simulink model "PILnewH"  (R2021a)
settings: Solver=FixedStepAuto  StartTime=0.0  StopTime=41.24  FixedStep=0.001  RelTol=1e-3  EnableMultiTasking=on
values from neighbouring files (symbols this model uses):
  den_lpf_d = den_lpf20    [Mainframe_init.m]    (also in load_autopilot.m)
  Emulated_FCC_IO_Delay = 7    [Mainframe_init.m]
  Enable_Gyros = 0    [Mainframe_init.m]
  Enable_INS = 0    [Mainframe_init.m]
  num_lpf_d = num_lpf20    [Mainframe_init.m]    (also in load_autopilot.m)
undefined symbols (not defined in the file or in its folder): act_dmp, act_omega, Actuator, Aerodynamics, aMode, Autopilot, AUX, c_b_WGS, c_be, c_flat, c_grav, c_h_geop0, c_h_geope, c_pa0, c_pe, c_r0, c_rot, c_rsma, c_Tmp0, d_siB_0, d_siB_max, d_siB_min, dd_siB_max, dd_siB_min, dev, DiscIntNeverNeededParam, e_pa, e_Tmp, Earth, fin_maxrate, flag_I_act_switch, flag_I_aero_switch, flag_I_flat, flag_I_gravity_switch, flag_I_rot, hcr, HIL_Data, JMMM_0, JMMM_e, JSPB_e, lat_0, lon_0, Mass_Props, mB_0, mM_0, mM_e, National_Instruments, pBII_0, PCIe, pMPB, pNPB, propellant_kg, prp_FBPB, prp_mdot, prp_T, pSPB, pwm_output1, qEG_0, qIB_0, qIE_0 ... (+29)
libraries: simulink x31, simulink_extras x24, aerolibcommonsys x4, px4lib x2, custom_blocks x1, pil_lib x1, aerolibtransform2 x1, sldrtlib x1, aerolibnav x1
(part 8 of 15)

== system PILnewH/Non-linear Flight Dynamic Model/GRM_Airframe/motion_kinematics/calc_motion_kinematics/earth_rotation/quaternion_integration ==
  wEIE : Inport
  Constant8 : Constant  Value=qIE_0
  Subsystem1 : Subsystem
  T12_from_q12 : Subsystem
      mask help: Transforms a quaternion into a Direction Cosine Matrix
      mask Help:
      | Name:
      | 
      |     T12_from_q12
      | 
      | Description:
      | 
      |     This block implements the transformation of a quaternion into the
      |     corresponding direction cosine matrix DCM.
      | 
      | Inputs  [size] [data type] [unit]:
      | 
      |     quaternion q12 [4] [double] [-]
      | 
      | Outputs  [size] [data type] [unit]:
      | 
      |     direction cosine matrix T12  [3x3] [double] [-]
      mask Display:
      | %port_label('input', 1, 'q12')
      | %port_label('output', 1, 'T12')
      | disp('q \rightarrow DCM','texmode','on')
  integration_eom : Integrator  InitialConditionSource=external
  qIE : Outport  VectorParamsAs1DForOutWhenUnconnected=off
  TIE : Outport  Port=2  VectorParamsAs1DForOutWhenUnconnected=off
  wires:
  Subsystem1/1(d_qIE) -> integration_eom/1
  integration_eom/1 -> qIE/1, Subsystem1/2(qIE), T12_from_q12/1(q12)  "qIE"
  wEIE/1 -> Subsystem1/1(wEIE)
  T12_from_q12/1(T12) -> TIE/1  "TIE"
  Constant8/1 -> integration_eom/2

== system PILnewH/Non-linear Flight Dynamic Model/GRM_Airframe/motion_kinematics/calc_motion_kinematics/earth_rotation/quaternion_integration1 ==
  wGEG : Inport
  Constant8 : Constant  Value=qEG_0
  Subsystem1 : Subsystem
  T12_from_q12 : Subsystem
      mask help: Transforms a quaternion into a Direction Cosine Matrix
      mask Help:
      | Name:
      | 
      |     T12_from_q12
      | 
      | Description:
      | 
      |     This block implements the transformation of a quaternion into the
      |     corresponding direction cosine matrix DCM.
      | 
      | Inputs  [size] [data type] [unit]:
      | 
      |     quaternion q12 [4] [double] [-]
      | 
      | Outputs  [size] [data type] [unit]:
      | 
      |     direction cosine matrix T12  [3x3] [double] [-]
      mask Display:
      | %port_label('input', 1, 'q12')
      | %port_label('output', 1, 'T12')
      | disp('q \rightarrow DCM','texmode','on')
  integration_eom : Integrator  InitialConditionSource=external
  qEG : Outport  VectorParamsAs1DForOutWhenUnconnected=off
  TEG : Outport  Port=2  VectorParamsAs1DForOutWhenUnconnected=off
  wires:
  Constant8/1 -> integration_eom/2
  T12_from_q12/1(T12) -> TEG/1  "TEG"
  wGEG/1 -> Subsystem1/1(wGEG)
  integration_eom/1 -> T12_from_q12/1(q12), Subsystem1/2(qEG), qEG/1  "qEG"
  Subsystem1/1(d_qEG) -> integration_eom/1

== system PILnewH/Non-linear Flight Dynamic Model/GRM_Airframe/motion_kinematics/calc_motion_kinematics/earth_rotation/transport_rate ==
  lat : Inport
  lon : Inport  Port=2
  Constant8 : Constant  Value=0
  Constant9 : Constant  Value=flag_I_flat
  Derivative : Derivative  CoefficientInTFapproximation=1
  Derivative1 : Derivative  CoefficientInTFapproximation=1
  Gain1 : Gain  Gain=-1
  Gain2 : Gain  Gain=-1
  Product : Product
  Product1 : Product
  Switch : Switch  Criteria=u2 > Threshold
  Trigonometric Function : Trigonometry
  Trigonometric Function1 : Trigonometry  Operator=cos
  Vector Concatenate : Concatenate  NumInputs=3
  Vector Concatenate1 : Concatenate  NumInputs=3
  wEGG : Outport  VectorParamsAs1DForOutWhenUnconnected=off
  wires:
  Derivative/1 -> Gain1/1
  Trigonometric Function/1 -> Product/1
  lat/1 -> Trigonometric Function1/1, Derivative/1, Trigonometric Function/1
  Derivative1/1 -> Product1/1, Product/2
  Product/1 -> Gain2/1
  Gain2/1 -> Vector Concatenate/3
  Gain1/1 -> Vector Concatenate/2
  Product1/1 -> Vector Concatenate/1
  Trigonometric Function1/1 -> Product1/2
  lon/1 -> Derivative1/1
  Vector Concatenate/1 -> Switch/3  "wEGG"
  Constant9/1 -> Switch/2
  Vector Concatenate1/1 -> Switch/1  "wEGG"
  Constant8/1 -> Vector Concatenate1/1, Vector Concatenate1/3, Vector Concatenate1/2
  Switch/1 -> wEGG/1  "wEGG"

== system PILnewH/Non-linear Flight Dynamic Model/GRM_Airframe/propulsion/prp_uncertainty/3_rot_mat/1. Rotation x-Achse ==
  alpha1 : Inport
  Constant : Constant
  Constant{1..2,7..8} (4 alike) : Constant  Value=0
  Gain : Gain  Gain=-1
  Matrix Concatenate : Concatenate  NumInputs=3  Mode=Multidimensional array  ConcatenateDimension=2
  Mux : Mux  Inputs=3
  Mux1 : Mux  Inputs=3
  Mux2 : Mux  Inputs=3
  Trigonometric Function : Trigonometry  Operator=cos
  Trigonometric Function1 : Trigonometry
  Trigonometric Function2 : Trigonometry
  Trigonometric Function3 : Trigonometry  Operator=cos
  1Rot_Matrix_x : Outport  VectorParamsAs1DForOutWhenUnconnected=off
  wires:
  Gain/1 -> Mux1/3
  alpha1/1 -> Trigonometric Function2/1, Trigonometric Function/1, Trigonometric Function1/1, Trigonometric Function3/1
  Constant/1 -> Mux/1
  Constant1/1 -> Mux/2
  Constant2/1 -> Mux/3
  Constant8/1 -> Mux1/1
  Trigonometric Function/1 -> Mux1/2
  Trigonometric Function2/1 -> Gain/1
  Constant7/1 -> Mux2/1
  Trigonometric Function1/1 -> Mux2/2
  Trigonometric Function3/1 -> Mux2/3
  Mux/1 -> Matrix Concatenate/1
  Mux1/1 -> Matrix Concatenate/2
  Mux2/1 -> Matrix Concatenate/3
  Matrix Concatenate/1 -> 1Rot_Matrix_x/1

== system PILnewH/Non-linear Flight Dynamic Model/GRM_Airframe/propulsion/prp_uncertainty/3_rot_mat/1. Rotation y-Achse ==
  alpha1 : Inport
  Constant{,2,7..8} (4 alike) : Constant  Value=0
  Constant1 : Constant
  Gain1 : Gain  Gain=-1
  Matrix Concatenate : Concatenate  NumInputs=3  Mode=Multidimensional array  ConcatenateDimension=2
  Mux : Mux  Inputs=3
  Mux1 : Mux  Inputs=3
  Mux2 : Mux  Inputs=3
  Trigonometric Function : Trigonometry  Operator=cos
  Trigonometric Function1 : Trigonometry
  Trigonometric Function2 : Trigonometry
  Trigonometric Function3 : Trigonometry  Operator=cos
  1Rot_Matrix_y : Outport  VectorParamsAs1DForOutWhenUnconnected=off
  wires:
  Gain1/1 -> Mux2/1
  Mux2/1 -> Matrix Concatenate/3
  Mux1/1 -> Matrix Concatenate/2
  Mux/1 -> Matrix Concatenate/1
  Trigonometric Function3/1 -> Mux2/3
  Trigonometric Function1/1 -> Gain1/1
  Constant2/1 -> Mux1/3
  Constant1/1 -> Mux1/2
  Constant/1 -> Mux1/1
  alpha1/1 -> Trigonometric Function1/1, Trigonometric Function3/1, Trigonometric Function2/1, Trigonometric Function/1
  Constant8/1 -> Mux/2
  Trigonometric Function/1 -> Mux/1
  Trigonometric Function2/1 -> Mux/3
  Constant7/1 -> Mux2/2
  Matrix Concatenate/1 -> 1Rot_Matrix_y/1

== system PILnewH/Non-linear Flight Dynamic Model/GRM_Airframe/propulsion/prp_uncertainty/3_rot_mat/1. Rotation z-Achse ==
  alpha1 : Inport
  Constant{4,7..8,10} (4 alike) : Constant  Value=0
  Constant11 : Constant
  Gain : Gain  Gain=-1
  Matrix Concatenate : Concatenate  NumInputs=3  Mode=Multidimensional array  ConcatenateDimension=2
  Mux : Mux  Inputs=3
  Mux1 : Mux  Inputs=3
  Mux2 : Mux  Inputs=3
  Trigonometric Function : Trigonometry  Operator=cos
  Trigonometric Function1 : Trigonometry
  Trigonometric Function3 : Trigonometry  Operator=cos
  Trigonometric Function4 : Trigonometry
  1Rot_Matrix_z : Outport  VectorParamsAs1DForOutWhenUnconnected=off
  wires:
  Gain/1 -> Mux/2
  Trigonometric Function/1 -> Mux1/2
  Mux/1 -> Matrix Concatenate/1
  Mux1/1 -> Matrix Concatenate/2
  Mux2/1 -> Matrix Concatenate/3
  Trigonometric Function1/1 -> Mux1/1
  Constant7/1 -> Mux1/3
  Constant4/1 -> Mux2/1
  Constant10/1 -> Mux2/2
  Constant11/1 -> Mux2/3
  Trigonometric Function3/1 -> Mux/1
  Trigonometric Function4/1 -> Gain/1
  Constant8/1 -> Mux/3
  Matrix Concatenate/1 -> 1Rot_Matrix_z/1
  alpha1/1 -> Trigonometric Function3/1, Trigonometric Function4/1, Trigonometric Function/1, Trigonometric Function1/1

== system PILnewH/Non-linear Flight Dynamic Model/GRM_Airframe/propulsion/prp_uncertainty/3_rot_mat/2. Rotation x-Achse ==
  alpha2 : Inport
  Constant : Constant
  Constant{1..2,7..8} (4 alike) : Constant  Value=0
  Gain : Gain  Gain=-1
  Matrix Concatenate : Concatenate  NumInputs=3  Mode=Multidimensional array  ConcatenateDimension=2
  Mux : Mux  Inputs=3
  Mux1 : Mux  Inputs=3
  Mux2 : Mux  Inputs=3
  Trigonometric Function : Trigonometry  Operator=cos
  Trigonometric Function1 : Trigonometry
  Trigonometric Function2 : Trigonometry
  Trigonometric Function3 : Trigonometry  Operator=cos
  2Rot_Matrix_x : Outport  VectorParamsAs1DForOutWhenUnconnected=off
  wires:
  Gain/1 -> Mux1/3
  alpha2/1 -> Trigonometric Function2/1, Trigonometric Function/1, Trigonometric Function1/1, Trigonometric Function3/1
  Constant/1 -> Mux/1
  Constant1/1 -> Mux/2
  Constant2/1 -> Mux/3
  Constant8/1 -> Mux1/1
  Trigonometric Function/1 -> Mux1/2
  Trigonometric Function2/1 -> Gain/1
  Constant7/1 -> Mux2/1
  Trigonometric Function1/1 -> Mux2/2
  Trigonometric Function3/1 -> Mux2/3
  Mux/1 -> Matrix Concatenate/1
  Mux1/1 -> Matrix Concatenate/2
  Mux2/1 -> Matrix Concatenate/3
  Matrix Concatenate/1 -> 2Rot_Matrix_x/1

== system PILnewH/Non-linear Flight Dynamic Model/GRM_Airframe/propulsion/prp_uncertainty/3_rot_mat/2. Rotation y-Achse ==
  alpha2 : Inport
  Constant{,2,7..8} (4 alike) : Constant  Value=0
  Constant1 : Constant
  Gain1 : Gain  Gain=-1
  Matrix Concatenate : Concatenate  NumInputs=3  Mode=Multidimensional array  ConcatenateDimension=2
  Mux : Mux  Inputs=3
  Mux1 : Mux  Inputs=3
  Mux2 : Mux  Inputs=3
  Trigonometric Function : Trigonometry  Operator=cos
  Trigonometric Function1 : Trigonometry
  Trigonometric Function2 : Trigonometry
  Trigonometric Function3 : Trigonometry  Operator=cos
  2Rot_Matrix_y : Outport  VectorParamsAs1DForOutWhenUnconnected=off
  wires:
  Gain1/1 -> Mux2/1
  Mux2/1 -> Matrix Concatenate/3
  Mux1/1 -> Matrix Concatenate/2
  Mux/1 -> Matrix Concatenate/1
  Trigonometric Function3/1 -> Mux2/3
  Trigonometric Function1/1 -> Gain1/1
  Constant2/1 -> Mux1/3
  Constant1/1 -> Mux1/2
  Constant/1 -> Mux1/1
  alpha2/1 -> Trigonometric Function1/1, Trigonometric Function3/1, Trigonometric Function2/1, Trigonometric Function/1
  Constant8/1 -> Mux/2
  Trigonometric Function/1 -> Mux/1
  Trigonometric Function2/1 -> Mux/3
  Constant7/1 -> Mux2/2
  Matrix Concatenate/1 -> 2Rot_Matrix_y/1

== system PILnewH/Non-linear Flight Dynamic Model/GRM_Airframe/propulsion/prp_uncertainty/3_rot_mat/2. Rotation z-Achse ==
  alpha2 : Inport
  Constant{4,7..8,10} (4 alike) : Constant  Value=0
  Constant11 : Constant
  Gain : Gain  Gain=-1
  Matrix Concatenate : Concatenate  NumInputs=3  Mode=Multidimensional array  ConcatenateDimension=2
  Mux : Mux  Inputs=3
  Mux1 : Mux  Inputs=3
  Mux2 : Mux  Inputs=3
  Trigonometric Function : Trigonometry  Operator=cos
  Trigonometric Function1 : Trigonometry
  Trigonometric Function3 : Trigonometry  Operator=cos
  Trigonometric Function4 : Trigonometry
  2Rot_Matrix_z : Outport  VectorParamsAs1DForOutWhenUnconnected=off
  wires:
  Gain/1 -> Mux/2
  Trigonometric Function/1 -> Mux1/2
  Mux/1 -> Matrix Concatenate/1
  Mux1/1 -> Matrix Concatenate/2
  Mux2/1 -> Matrix Concatenate/3
  Trigonometric Function1/1 -> Mux1/1
  Constant7/1 -> Mux1/3
  Constant4/1 -> Mux2/1
  Constant10/1 -> Mux2/2
  Constant11/1 -> Mux2/3
  Trigonometric Function3/1 -> Mux/1
  Trigonometric Function4/1 -> Gain/1
  Constant8/1 -> Mux/3
  Matrix Concatenate/1 -> 2Rot_Matrix_z/1
  alpha2/1 -> Trigonometric Function3/1, Trigonometric Function4/1, Trigonometric Function/1, Trigonometric Function1/1

== system PILnewH/Non-linear Flight Dynamic Model/GRM_Airframe/propulsion/prp_uncertainty/3_rot_mat/3. Rotation x-Achse ==
  alpha3 : Inport
  Constant : Constant
  Constant{1..2,7..8} (4 alike) : Constant  Value=0
  Gain : Gain  Gain=-1
  Matrix Concatenate : Concatenate  NumInputs=3  Mode=Multidimensional array  ConcatenateDimension=2
  Mux : Mux  Inputs=3
  Mux1 : Mux  Inputs=3
  Mux2 : Mux  Inputs=3
  Trigonometric Function : Trigonometry  Operator=cos
  Trigonometric Function1 : Trigonometry
  Trigonometric Function2 : Trigonometry
  Trigonometric Function3 : Trigonometry  Operator=cos
  3Rot_Matrix_x : Outport  VectorParamsAs1DForOutWhenUnconnected=off
  wires:
  Gain/1 -> Mux1/3
  alpha3/1 -> Trigonometric Function2/1, Trigonometric Function/1, Trigonometric Function1/1, Trigonometric Function3/1
  Constant/1 -> Mux/1
  Constant1/1 -> Mux/2
  Constant2/1 -> Mux/3
  Constant8/1 -> Mux1/1
  Trigonometric Function/1 -> Mux1/2
  Trigonometric Function2/1 -> Gain/1
  Constant7/1 -> Mux2/1
  Trigonometric Function1/1 -> Mux2/2
  Trigonometric Function3/1 -> Mux2/3
  Mux/1 -> Matrix Concatenate/1
  Mux1/1 -> Matrix Concatenate/2
  Mux2/1 -> Matrix Concatenate/3
  Matrix Concatenate/1 -> 3Rot_Matrix_x/1

== system PILnewH/Non-linear Flight Dynamic Model/GRM_Airframe/propulsion/prp_uncertainty/3_rot_mat/3. Rotation y-Achse ==
  alpha3 : Inport
  Constant{,2,7..8} (4 alike) : Constant  Value=0
  Constant1 : Constant
  Gain1 : Gain  Gain=-1
  Matrix Concatenate : Concatenate  NumInputs=3  Mode=Multidimensional array  ConcatenateDimension=2
  Mux : Mux  Inputs=3
  Mux1 : Mux  Inputs=3
  Mux2 : Mux  Inputs=3
  Trigonometric Function : Trigonometry  Operator=cos
  Trigonometric Function1 : Trigonometry
  Trigonometric Function2 : Trigonometry
  Trigonometric Function3 : Trigonometry  Operator=cos
  3Rot_Matrix_y : Outport  VectorParamsAs1DForOutWhenUnconnected=off
  wires:
  Gain1/1 -> Mux2/1
  Mux2/1 -> Matrix Concatenate/3
  Mux1/1 -> Matrix Concatenate/2
  Mux/1 -> Matrix Concatenate/1
  Trigonometric Function3/1 -> Mux2/3
  Trigonometric Function1/1 -> Gain1/1
  Constant2/1 -> Mux1/3
  Constant1/1 -> Mux1/2
  Constant/1 -> Mux1/1
  alpha3/1 -> Trigonometric Function1/1, Trigonometric Function3/1, Trigonometric Function2/1, Trigonometric Function/1
  Constant8/1 -> Mux/2
  Trigonometric Function/1 -> Mux/1
  Trigonometric Function2/1 -> Mux/3
  Constant7/1 -> Mux2/2
  Matrix Concatenate/1 -> 3Rot_Matrix_y/1

== system PILnewH/Non-linear Flight Dynamic Model/GRM_Airframe/propulsion/prp_uncertainty/3_rot_mat/3. Rotation z-Achse ==
  alpha3 : Inport
  Constant{4,7..8,10} (4 alike) : Constant  Value=0
  Constant11 : Constant
  Gain : Gain  Gain=-1
  Matrix Concatenate : Concatenate  NumInputs=3  Mode=Multidimensional array  ConcatenateDimension=2
  Mux : Mux  Inputs=3
  Mux1 : Mux  Inputs=3
  Mux2 : Mux  Inputs=3
  Trigonometric Function : Trigonometry  Operator=cos
  Trigonometric Function1 : Trigonometry
  Trigonometric Function3 : Trigonometry  Operator=cos
  Trigonometric Function4 : Trigonometry
  3Rot_Matrix_z : Outport  VectorParamsAs1DForOutWhenUnconnected=off
  wires:
  Gain/1 -> Mux/2
  Trigonometric Function/1 -> Mux1/2
  Mux/1 -> Matrix Concatenate/1
  Mux1/1 -> Matrix Concatenate/2
  Mux2/1 -> Matrix Concatenate/3
  Trigonometric Function1/1 -> Mux1/1
  Constant7/1 -> Mux1/3
  Constant4/1 -> Mux2/1
  Constant10/1 -> Mux2/2
  Constant11/1 -> Mux2/3
  Trigonometric Function3/1 -> Mux/1
  Trigonometric Function4/1 -> Gain/1
  Constant8/1 -> Mux/3
  Matrix Concatenate/1 -> 3Rot_Matrix_z/1
  alpha3/1 -> Trigonometric Function3/1, Trigonometric Function4/1, Trigonometric Function/1, Trigonometric Function1/1

== system PILnewH/Non-linear Flight Dynamic Model/GRM_Airframe/rb_eom/calc_bus_flight_dyn_bus_entries/Subsystem2/trafo_E_to_geodetic ==
  note: Outputs [size]:
      |
      | geodetic longitude [1]
      | geodetic latitude [1]
      | geodetic altitude [1]
  note: Inputs [size]:
      |
      | position_E [3]
  pBEE : Inport
  Geodetic_altitude : Subsystem
  Geodetic_latitude : Subsystem
  Selector1 : Selector  IndexMode=Zero-based  InputPortWidth=3  IndexOptions=Index vector (dialog)  Indices=1  OutputSizes=1
  Selector2 : Selector  IndexMode=Zero-based  InputPortWidth=3  IndexOptions=Index vector (dialog)  Indices=0  OutputSizes=1
  Trigonometric Function1 : Trigonometry  Operator=atan2
  c_flat : Constant  Value=c_flat
  c_rsma : Constant  Value=c_rsma
  lon : Outport  VectorParamsAs1DForOutWhenUnconnected=off
  lat : Outport  Port=2  VectorParamsAs1DForOutWhenUnconnected=off
  alt : Outport  Port=3  VectorParamsAs1DForOutWhenUnconnected=off
  wires:
  c_flat/1 -> Geodetic_altitude/3(c_flat), Geodetic_latitude/3(c_flat)  "c_flat"
  c_rsma/1 -> Geodetic_latitude/2(c_rsma), Geodetic_altitude/2(c_rsma)  "c_rsma"
  Selector1/1 -> Trigonometric Function1/1  "pBEE_y"
  Selector2/1 -> Trigonometric Function1/2  "pBEE_x"
  Geodetic_latitude/1(lat) -> Geodetic_altitude/4(lat), lat/1
  Geodetic_altitude/1(alt) -> alt/1
  Trigonometric Function1/1 -> lon/1  "lon"
  pBEE/1 -> Selector1/1, Selector2/1, Geodetic_latitude/1(pBEE), Geodetic_altitude/1(pBEE)  "pBEE"

== system PILnewH/Non-linear Flight Dynamic Model/GRM_Airframe/rb_eom/calc_bus_flight_dyn_bus_entries/q12_from_T12/Case 0 ==
  dcm11 : Inport
  dcm22 : Inport  Port=2
  dcm33 : Inport  Port=3
  Add : Sum
  Add1 : Sum
  Add2 : Sum
  Logical Operator : Logic  Inputs=3  AllPortsSameDT=off  OutDataTypeStr=boolean
  dcm11 >= -dcm22 : simulink/Logic and Bit Operations/Compare To Zero  relop=>=  OutDataTypeStr=boolean
      settings: SourceProductName=ISim Simulink Block Set
  dcm11 >= -dcm33 : simulink/Logic and Bit Operations/Compare To Zero  relop=>=  OutDataTypeStr=boolean
      settings: SourceProductName=ISim Simulink Block Set
  dcm22 >= -dcm33 : simulink/Logic and Bit Operations/Compare To Zero  relop=>=  OutDataTypeStr=boolean
      settings: SourceProductName=ISim Simulink Block Set
  q_R^0(R) : Outport  VectorParamsAs1DForOutWhenUnconnected=off
  wires:
  Logical Operator/1 -> q_R^0(R)/1  "q_R^0(R)"
  dcm22 >= -dcm33/1 -> Logical Operator/3
  dcm11/1 -> Add/1, Add1/1
  dcm11 >= -dcm33/1 -> Logical Operator/2
  dcm11 >= -dcm22/1 -> Logical Operator/1
  Add2/1 -> dcm22 >= -dcm33/1
  Add1/1 -> dcm11 >= -dcm33/1
  Add/1 -> dcm11 >= -dcm22/1
  dcm33/1 -> Add1/2, Add2/2
  dcm22/1 -> Add/2, Add2/1

== system PILnewH/Non-linear Flight Dynamic Model/GRM_Airframe/rb_eom/calc_bus_flight_dyn_bus_entries/q12_from_T12/Case 1 ==
  dcm11 : Inport
  dcm22 : Inport  Port=2
  dcm33 : Inport  Port=3
  Add : Sum  Inputs=+-
  Add1 : Sum  Inputs=+-
  Add2 : Sum
  Logical Operator : Logic  Inputs=3  AllPortsSameDT=off  OutDataTypeStr=boolean
  dcm11 >= dcm22 : simulink/Logic and Bit Operations/Compare To Zero  relop=>=  OutDataTypeStr=boolean
      settings: SourceProductName=ISim Simulink Block Set
  dcm11 >= dcm33 : simulink/Logic and Bit Operations/Compare To Zero  relop=>=  OutDataTypeStr=boolean
      settings: SourceProductName=ISim Simulink Block Set
  dcm22 < -dcm33 : simulink/Logic and Bit Operations/Compare To Zero  relop=<  OutDataTypeStr=boolean
      settings: SourceProductName=ISim Simulink Block Set
  q_R^1(R) : Outport  VectorParamsAs1DForOutWhenUnconnected=off
  wires:
  Logical Operator/1 -> q_R^1(R)/1  "q_R^1(R)"
  dcm22 < -dcm33/1 -> Logical Operator/3
  dcm11/1 -> Add/1, Add1/1
  dcm11 >= dcm33/1 -> Logical Operator/2
  dcm11 >= dcm22/1 -> Logical Operator/1
  Add2/1 -> dcm22 < -dcm33/1
  Add1/1 -> dcm11 >= dcm33/1
  Add/1 -> dcm11 >= dcm22/1
  dcm33/1 -> Add1/2, Add2/2
  dcm22/1 -> Add/2, Add2/1

== system PILnewH/Non-linear Flight Dynamic Model/GRM_Airframe/rb_eom/calc_bus_flight_dyn_bus_entries/q12_from_T12/Case 2 ==
  dcm11 : Inport
  dcm22 : Inport  Port=2
  dcm33 : Inport  Port=3
  Add : Sum  Inputs=+-
  Add1 : Sum
  Add2 : Sum  Inputs=+-
  Logical Operator : Logic  Inputs=3  AllPortsSameDT=off  OutDataTypeStr=boolean
  dcm11 < -dcm33 : simulink/Logic and Bit Operations/Compare To Zero  relop=<  OutDataTypeStr=boolean
      settings: SourceProductName=ISim Simulink Block Set
  dcm11 < dcm22 : simulink/Logic and Bit Operations/Compare To Zero  relop=<  OutDataTypeStr=boolean
      settings: SourceProductName=ISim Simulink Block Set
  dcm22 >= dcm33 : simulink/Logic and Bit Operations/Compare To Zero  relop=>=  OutDataTypeStr=boolean
      settings: SourceProductName=ISim Simulink Block Set
  q_R^2(R) : Outport  VectorParamsAs1DForOutWhenUnconnected=off
  wires:
  Logical Operator/1 -> q_R^2(R)/1  "q_R^2(R)"
  dcm22 >= dcm33/1 -> Logical Operator/3
  dcm11/1 -> Add/1, Add1/1
  dcm11 < -dcm33/1 -> Logical Operator/2
  dcm11 < dcm22/1 -> Logical Operator/1
  Add2/1 -> dcm22 >= dcm33/1
  Add1/1 -> dcm11 < -dcm33/1
  Add/1 -> dcm11 < dcm22/1
  dcm33/1 -> Add1/2, Add2/2
  dcm22/1 -> Add/2, Add2/1

== system PILnewH/Non-linear Flight Dynamic Model/GRM_Airframe/rb_eom/calc_bus_flight_dyn_bus_entries/q12_from_T12/Case 3 ==
  dcm11 : Inport
  dcm22 : Inport  Port=2
  dcm33 : Inport  Port=3
  Add : Sum
  Add1 : Sum  Inputs=+-
  Add2 : Sum  Inputs=+-
  Logical Operator : Logic  Inputs=3  AllPortsSameDT=off  OutDataTypeStr=boolean
  dcm11 < -dcm22 : simulink/Logic and Bit Operations/Compare To Zero  relop=<  OutDataTypeStr=boolean
      settings: SourceProductName=ISim Simulink Block Set
  dcm11 < dcm33 : simulink/Logic and Bit Operations/Compare To Zero  relop=<  OutDataTypeStr=boolean
      settings: SourceProductName=ISim Simulink Block Set
  dcm22 < dcm33 : simulink/Logic and Bit Operations/Compare To Zero  relop=<  OutDataTypeStr=boolean
      settings: SourceProductName=ISim Simulink Block Set
  q_R^3(R) : Outport  VectorParamsAs1DForOutWhenUnconnected=off
  wires:
  Logical Operator/1 -> q_R^3(R)/1  "q_R^3(R)"
  dcm22 < dcm33/1 -> Logical Operator/3
  dcm11/1 -> Add/1, Add1/1
  dcm11 < dcm33/1 -> Logical Operator/2
  dcm11 < -dcm22/1 -> Logical Operator/1
  Add2/1 -> dcm22 < dcm33/1
  Add1/1 -> dcm11 < dcm33/1
  Add/1 -> dcm11 < -dcm22/1
  dcm33/1 -> Add1/2, Add2/2
  dcm22/1 -> Add/2, Add2/1

== system PILnewH/Non-linear Flight Dynamic Model/GRM_Airframe/rb_eom/calc_bus_flight_dyn_bus_entries/q12_from_T12/normalize_quaternion ==
  note: Outputs [size]:
      |
      | q_norm [4x1]
  note: Inputs [size]:
      |
      | q [4x1]
  q : Inport  PortDimensions=[4 1]
  Add : Sum  Inputs=++++
  Demux : Demux  Outputs=[1;1;1;1]
  Math Function : Math  Operator=sqrt  SignedPower=on  SaturateOnIntegerOverflow=on
  Product : Product  Inputs=*/  InputSameDT=on  RndMeth=Zero  SaturateOnIntegerOverflow=on  OutDataTypeStr=Inherit: Same as first input
  Product{1..4} (4 alike) : Product  RndMeth=Zero
  q_normalized : Outport  PortDimensions=[4 1]  VectorParamsAs1DForOutWhenUnconnected=off
  wires:
  Math Function/1 -> Product/2
  Add/1 -> Math Function/1
  Product1/1 -> Add/1
  Product2/1 -> Add/2
  Product3/1 -> Add/3
  Product4/1 -> Add/4
  Demux/4 -> Product4/2, Product4/1
  Demux/3 -> Product3/2, Product3/1
  Demux/2 -> Product2/2, Product2/1
  Demux/1 -> Product1/2, Product1/1
  q/1 -> Demux/1, Product/1
  Product/1 -> q_normalized/1

== system PILnewH/Non-linear Flight Dynamic Model/GRM_Airframe/rb_eom/calc_bus_flight_dyn_bus_entries/q12_from_T12/q_R^0(R) ==
  DCM : Inport
  q_R^0(R) = TRUE : EnablePort
  (1+r11+r22+r33)^1/2 : Sqrt  SaturateOnIntegerOverflow=on
  Add : Sum  Inputs=++++
  Constant : Constant
  Divide : Product  Inputs=*/
  Divide1 : Product  Inputs=*/
  Divide2 : Product  Inputs=*/
  Gain : Gain  Gain=0.5
  Saturation : Saturate  UpperLimit=inf  LowerLimit=eps
      settings: AttributesFormatString=|
      | %<UpperLimit>
      | %<LowerLimit>
  Subtract : Sum  Inputs=+-
  Subtract1 : Sum  Inputs=+-
  Subtract2 : Sum  Inputs=+-
  Vector Concatenate : Concatenate  NumInputs=4
  dcm11 : Selector  NumberOfDimensions=2  IndexMode=Zero-based  InputPortWidth=3  IndexOptions=Index vector (dialog),Index vector (dialog)  Indices=0,0  OutputSizes=1,1
  dcm12 : Selector  NumberOfDimensions=2  IndexMode=Zero-based  InputPortWidth=3  IndexOptions=Index vector (dialog),Index vector (dialog)  Indices=0,1  OutputSizes=1,1
  dcm13 : Selector  NumberOfDimensions=2  IndexMode=Zero-based  InputPortWidth=3  IndexOptions=Index vector (dialog),Index vector (dialog)  Indices=0,2  OutputSizes=1,1
  dcm21 : Selector  NumberOfDimensions=2  IndexMode=Zero-based  InputPortWidth=3  IndexOptions=Index vector (dialog),Index vector (dialog)  Indices=1,0  OutputSizes=1,1
  dcm22 : Selector  NumberOfDimensions=2  IndexMode=Zero-based  InputPortWidth=3  IndexOptions=Index vector (dialog),Index vector (dialog)  Indices=1,1  OutputSizes=1,1
  dcm23 : Selector  NumberOfDimensions=2  IndexMode=Zero-based  InputPortWidth=3  IndexOptions=Index vector (dialog),Index vector (dialog)  Indices=1,2  OutputSizes=1,1
  dcm31 : Selector  NumberOfDimensions=2  IndexMode=Zero-based  InputPortWidth=3  IndexOptions=Index vector (dialog),Index vector (dialog)  Indices=2,0  OutputSizes=1,1
  dcm32 : Selector  NumberOfDimensions=2  IndexMode=Zero-based  InputPortWidth=3  IndexOptions=Index vector (dialog),Index vector (dialog)  Indices=2,1  OutputSizes=1,1
  dcm33 : Selector  NumberOfDimensions=2  IndexMode=Zero-based  InputPortWidth=3  IndexOptions=Index vector (dialog),Index vector (dialog)  Indices=2,2  OutputSizes=1,1
  q_R^0(R) : Outport  VectorParamsAs1DForOutWhenUnconnected=off
  wires:
  Saturation/1 -> Divide/2, Divide1/2, Divide2/2, Vector Concatenate/4  "q4"
  Gain/1 -> q_R^0(R)/1
  Vector Concatenate/1 -> Gain/1
  Divide/1 -> Vector Concatenate/3  "q3"
  Divide1/1 -> Vector Concatenate/2  "q2"
  Divide2/1 -> Vector Concatenate/1  "q1"
  (1+r11+r22+r33)^1/2/1 -> Saturation/1
  Subtract/1 -> Divide2/1  "dcm23-dcm32"
  Subtract2/1 -> Divide1/1  "dcm31-dcm13"
  Subtract1/1 -> Divide/1  "dcm12-dcm21"
  dcm12/1 -> Subtract1/1  "dcm12"
  dcm21/1 -> Subtract1/2  "dcm21"
  dcm13/1 -> Subtract2/2  "dcm13"
  dcm31/1 -> Subtract2/1  "dcm31"
  dcm32/1 -> Subtract/2  "dcm32"
  dcm23/1 -> Subtract/1  "dcm23"
  Add/1 -> (1+r11+r22+r33)^1/2/1
  dcm33/1 -> Add/4  "dcm33"
  dcm22/1 -> Add/3  "dcm22"
  dcm11/1 -> Add/2  "dcm11"
  Constant/1 -> Add/1
  DCM/1 -> dcm12/1, dcm11/1, dcm22/1, dcm33/1, dcm21/1, dcm13/1, dcm31/1, dcm23/1, dcm32/1

== system PILnewH/Non-linear Flight Dynamic Model/GRM_Airframe/rb_eom/calc_bus_flight_dyn_bus_entries/q12_from_T12/q_R^1(R) ==
  DCM : Inport
  q_R^1(R) = TRUE : EnablePort
  (1+r11-r22-r33)^1/2 : Sqrt  SaturateOnIntegerOverflow=on
  Add : Sum  Inputs=++--
  Constant : Constant
  Divide : Product  Inputs=*/
  Divide1 : Product  Inputs=*/
  Divide2 : Product  Inputs=*/
  Gain : Gain  Gain=0.5
  Saturation : Saturate  UpperLimit=inf  LowerLimit=eps
      settings: AttributesFormatString=|
      | %<UpperLimit>
      | %<LowerLimit>
  Subtract : Sum  Inputs=+-
  Subtract1 : Sum
  Subtract2 : Sum
  Vector Concatenate : Concatenate  NumInputs=4
  dcm11 : Selector  NumberOfDimensions=2  IndexMode=Zero-based  InputPortWidth=3  IndexOptions=Index vector (dialog),Index vector (dialog)  Indices=0,0  OutputSizes=1,1
  dcm12 : Selector  NumberOfDimensions=2  IndexMode=Zero-based  InputPortWidth=3  IndexOptions=Index vector (dialog),Index vector (dialog)  Indices=0,1  OutputSizes=1,1
  dcm13 : Selector  NumberOfDimensions=2  IndexMode=Zero-based  InputPortWidth=3  IndexOptions=Index vector (dialog),Index vector (dialog)  Indices=0,2  OutputSizes=1,1
  dcm21 : Selector  NumberOfDimensions=2  IndexMode=Zero-based  InputPortWidth=3  IndexOptions=Index vector (dialog),Index vector (dialog)  Indices=1,0  OutputSizes=1,1
  dcm22 : Selector  NumberOfDimensions=2  IndexMode=Zero-based  InputPortWidth=3  IndexOptions=Index vector (dialog),Index vector (dialog)  Indices=1,1  OutputSizes=1,1
  dcm23 : Selector  NumberOfDimensions=2  IndexMode=Zero-based  InputPortWidth=3  IndexOptions=Index vector (dialog),Index vector (dialog)  Indices=1,2  OutputSizes=1,1
  dcm31 : Selector  NumberOfDimensions=2  IndexMode=Zero-based  InputPortWidth=3  IndexOptions=Index vector (dialog),Index vector (dialog)  Indices=2,0  OutputSizes=1,1
  dcm32 : Selector  NumberOfDimensions=2  IndexMode=Zero-based  InputPortWidth=3  IndexOptions=Index vector (dialog),Index vector (dialog)  Indices=2,1  OutputSizes=1,1
  dcm33 : Selector  NumberOfDimensions=2  IndexMode=Zero-based  InputPortWidth=3  IndexOptions=Index vector (dialog),Index vector (dialog)  Indices=2,2  OutputSizes=1,1
  q_R^1(R) : Outport  VectorParamsAs1DForOutWhenUnconnected=off
  wires:
  Saturation/1 -> Divide/2, Divide1/2, Divide2/2, Vector Concatenate/1  "q1"
  Gain/1 -> q_R^1(R)/1
  Vector Concatenate/1 -> Gain/1
  Divide/1 -> Vector Concatenate/2  "q2"
  Divide1/1 -> Vector Concatenate/3  "q3"
  Divide2/1 -> Vector Concatenate/4  "q4"
  (1+r11-r22-r33)^1/2/1 -> Saturation/1
  Subtract/1 -> Divide2/1  "dcm23-dcm32"
  Subtract2/1 -> Divide1/1  "dcm31+dcm13"
  Subtract1/1 -> Divide/1  "dcm12+dcm21"
  dcm12/1 -> Subtract1/1  "dcm12"
  dcm21/1 -> Subtract1/2  "dcm21"
  dcm13/1 -> Subtract2/2  "dcm13"
  dcm31/1 -> Subtract2/1  "dcm31"
  dcm32/1 -> Subtract/2  "dcm32"
  dcm23/1 -> Subtract/1  "dcm23"
  Add/1 -> (1+r11-r22-r33)^1/2/1
  dcm33/1 -> Add/4  "dcm33"
  dcm22/1 -> Add/3  "dcm22"
  dcm11/1 -> Add/2  "dcm11"
  Constant/1 -> Add/1
  DCM/1 -> dcm31/1, dcm13/1, dcm23/1, dcm32/1, dcm21/1, dcm12/1, dcm33/1, dcm22/1, dcm11/1

== system PILnewH/Non-linear Flight Dynamic Model/GRM_Airframe/rb_eom/calc_bus_flight_dyn_bus_entries/q12_from_T12/q_R^2(R) ==
  DCM : Inport
  q_R^2(R) = TRUE : EnablePort
  (1-r11+r22-r33)^1/2 : Sqrt  SaturateOnIntegerOverflow=on
  Add : Sum  Inputs=+-+-
  Constant : Constant
  Divide : Product  Inputs=*/
  Divide1 : Product  Inputs=*/
  Divide2 : Product  Inputs=*/
  Gain : Gain  Gain=0.5
  Saturation : Saturate  UpperLimit=inf  LowerLimit=eps
      settings: AttributesFormatString=|
      | %<UpperLimit>
      | %<LowerLimit>
  Subtract : Sum
  Subtract1 : Sum
  Subtract2 : Sum  Inputs=+-
  Vector Concatenate : Concatenate  NumInputs=4
  dcm11 : Selector  NumberOfDimensions=2  IndexMode=Zero-based  InputPortWidth=3  IndexOptions=Index vector (dialog),Index vector (dialog)  Indices=0,0  OutputSizes=1,1
  dcm12 : Selector  NumberOfDimensions=2  IndexMode=Zero-based  InputPortWidth=3  IndexOptions=Index vector (dialog),Index vector (dialog)  Indices=0,1  OutputSizes=1,1
  dcm13 : Selector  NumberOfDimensions=2  IndexMode=Zero-based  InputPortWidth=3  IndexOptions=Index vector (dialog),Index vector (dialog)  Indices=0,2  OutputSizes=1,1
  dcm21 : Selector  NumberOfDimensions=2  IndexMode=Zero-based  InputPortWidth=3  IndexOptions=Index vector (dialog),Index vector (dialog)  Indices=1,0  OutputSizes=1,1
  dcm22 : Selector  NumberOfDimensions=2  IndexMode=Zero-based  InputPortWidth=3  IndexOptions=Index vector (dialog),Index vector (dialog)  Indices=1,1  OutputSizes=1,1
  dcm23 : Selector  NumberOfDimensions=2  IndexMode=Zero-based  InputPortWidth=3  IndexOptions=Index vector (dialog),Index vector (dialog)  Indices=1,2  OutputSizes=1,1
  dcm31 : Selector  NumberOfDimensions=2  IndexMode=Zero-based  InputPortWidth=3  IndexOptions=Index vector (dialog),Index vector (dialog)  Indices=2,0  OutputSizes=1,1
  dcm32 : Selector  NumberOfDimensions=2  IndexMode=Zero-based  InputPortWidth=3  IndexOptions=Index vector (dialog),Index vector (dialog)  Indices=2,1  OutputSizes=1,1
  dcm33 : Selector  NumberOfDimensions=2  IndexMode=Zero-based  InputPortWidth=3  IndexOptions=Index vector (dialog),Index vector (dialog)  Indices=2,2  OutputSizes=1,1
  q_R^2(R) : Outport  VectorParamsAs1DForOutWhenUnconnected=off
  wires:
  Saturation/1 -> Divide1/2, Divide2/2, Divide/2, Vector Concatenate/2  "q2"
  Gain/1 -> q_R^2(R)/1
  Vector Concatenate/1 -> Gain/1
  (1-r11+r22-r33)^1/2/1 -> Saturation/1
  Divide2/1 -> Vector Concatenate/3  "q3"
  Divide1/1 -> Vector Concatenate/4  "q4"
  Divide/1 -> Vector Concatenate/1  "q1"
  Subtract/1 -> Divide2/1  "dcm23+dcm32"
  Subtract2/1 -> Divide1/1  "dcm31-dcm13"
  Subtract1/1 -> Divide/1  "dcm12+dcm21"
  dcm12/1 -> Subtract1/1  "dcm12"
  dcm21/1 -> Subtract1/2  "dcm21"
  dcm13/1 -> Subtract2/2  "dcm13"
  dcm31/1 -> Subtract2/1  "dcm31"
  dcm32/1 -> Subtract/2  "dcm32"
  dcm23/1 -> Subtract/1  "dcm23"
  Add/1 -> (1-r11+r22-r33)^1/2/1
  dcm33/1 -> Add/4  "dcm33"
  dcm22/1 -> Add/3  "dcm22"
  dcm11/1 -> Add/2  "dcm11"
  Constant/1 -> Add/1
  DCM/1 -> dcm23/1, dcm32/1, dcm31/1, dcm13/1, dcm33/1, dcm22/1, dcm11/1, dcm21/1, dcm12/1

== system PILnewH/Non-linear Flight Dynamic Model/GRM_Airframe/rb_eom/calc_bus_flight_dyn_bus_entries/q12_from_T12/q_R^3(R) ==
  DCM : Inport
  q_R^3(R) = TRUE : EnablePort
  (1-r11-r22+r33)^1/2 : Sqrt  SaturateOnIntegerOverflow=on
  Add : Sum  Inputs=+--+
  Constant : Constant
  Divide : Product  Inputs=*/
  Divide1 : Product  Inputs=*/
  Divide2 : Product  Inputs=*/
  Gain : Gain  Gain=0.5
  Saturation : Saturate  UpperLimit=inf  LowerLimit=eps
      settings: AttributesFormatString=|
      | %<UpperLimit>
      | %<LowerLimit>
  Subtract : Sum
  Subtract1 : Sum  Inputs=+-
  Subtract2 : Sum
  Vector Concatenate : Concatenate  NumInputs=4
  dcm11 : Selector  NumberOfDimensions=2  IndexMode=Zero-based  InputPortWidth=3  IndexOptions=Index vector (dialog),Index vector (dialog)  Indices=0,0  OutputSizes=1,1
  dcm12 : Selector  NumberOfDimensions=2  IndexMode=Zero-based  InputPortWidth=3  IndexOptions=Index vector (dialog),Index vector (dialog)  Indices=0,1  OutputSizes=1,1
  dcm13 : Selector  NumberOfDimensions=2  IndexMode=Zero-based  InputPortWidth=3  IndexOptions=Index vector (dialog),Index vector (dialog)  Indices=0,2  OutputSizes=1,1
  dcm21 : Selector  NumberOfDimensions=2  IndexMode=Zero-based  InputPortWidth=3  IndexOptions=Index vector (dialog),Index vector (dialog)  Indices=1,0  OutputSizes=1,1
  dcm22 : Selector  NumberOfDimensions=2  IndexMode=Zero-based  InputPortWidth=3  IndexOptions=Index vector (dialog),Index vector (dialog)  Indices=1,1  OutputSizes=1,1
  dcm23 : Selector  NumberOfDimensions=2  IndexMode=Zero-based  InputPortWidth=3  IndexOptions=Index vector (dialog),Index vector (dialog)  Indices=1,2  OutputSizes=1,1
  dcm31 : Selector  NumberOfDimensions=2  IndexMode=Zero-based  InputPortWidth=3  IndexOptions=Index vector (dialog),Index vector (dialog)  Indices=2,0  OutputSizes=1,1
  dcm32 : Selector  NumberOfDimensions=2  IndexMode=Zero-based  InputPortWidth=3  IndexOptions=Index vector (dialog),Index vector (dialog)  Indices=2,1  OutputSizes=1,1
  dcm33 : Selector  NumberOfDimensions=2  IndexMode=Zero-based  InputPortWidth=3  IndexOptions=Index vector (dialog),Index vector (dialog)  Indices=2,2  OutputSizes=1,1
  q_R^3(R) : Outport  VectorParamsAs1DForOutWhenUnconnected=off
  wires:
  Saturation/1 -> Divide1/2, Divide2/2, Vector Concatenate/3, Divide/2  "q3"
  Gain/1 -> q_R^3(R)/1
  Divide/1 -> Vector Concatenate/4  "q4"
  Vector Concatenate/1 -> Gain/1
  (1-r11-r22+r33)^1/2/1 -> Saturation/1
  Divide2/1 -> Vector Concatenate/2  "q2"
  Divide1/1 -> Vector Concatenate/1  "q1"
  Subtract/1 -> Divide2/1  "dcm23+dcm32"
  Subtract2/1 -> Divide1/1  "dcm31+dcm13"
  Subtract1/1 -> Divide/1  "dcm12-dcm21"
  dcm12/1 -> Subtract1/1  "dcm12"
  dcm21/1 -> Subtract1/2  "dcm21"
  dcm13/1 -> Subtract2/2  "dcm13"
  dcm31/1 -> Subtract2/1  "dcm31"
  dcm32/1 -> Subtract/2  "dcm32"
  dcm23/1 -> Subtract/1  "dcm23"
  Add/1 -> (1-r11-r22+r33)^1/2/1
  dcm33/1 -> Add/4  "dcm33"
  dcm22/1 -> Add/3  "dcm22"
  dcm11/1 -> Add/2  "dcm11"
  Constant/1 -> Add/1
  DCM/1 -> dcm13/1, dcm31/1, dcm23/1, dcm32/1, dcm11/1, dcm22/1, dcm33/1, dcm21/1, dcm12/1

== system PILnewH/Non-linear Flight Dynamic Model/GRM_Airframe/rb_eom/eom_6dof/Rigid_Body_EOM_6_DOF/Integration ==
  d_pBII : Inport
  d_vBII : Inport  Port=2
  d_qIB : Inport  Port=3
  d_wBIB : Inport  Port=4
  x0 : Inport  Port=5
  Bus Creator : BusCreator  Inputs=6
  Reshape : Reshape  OutputDimensionality=Customize  OutputDimensions=[13,1]
  Reshape1 : Reshape  OutputDimensionality=Customize  OutputDimensions=[3,1]
  Reshape2 : Reshape  OutputDimensionality=Customize  OutputDimensions=[3,1]
  Selector : Selector  IndexMode=Zero-based  InputPortWidth=13  IndexOptions=Index vector (dialog)  Indices=0:2  OutputSizes=3
  Selector1 : Selector  IndexMode=Zero-based  InputPortWidth=13  IndexOptions=Index vector (dialog)  Indices=3:5  OutputSizes=3
  Selector2 : Selector  IndexMode=Zero-based  InputPortWidth=13  IndexOptions=Index vector (dialog)  Indices=6:9  OutputSizes=3
  Selector3 : Selector  IndexMode=Zero-based  InputPortWidth=13  IndexOptions=Index vector (dialog)  Indices=10:12  OutputSizes=3
  Vector Concatenate : Concatenate  NumInputs=4  ConcatenateDimension=2
  integration_eom : Integrator  InitialConditionSource=external
  normalize_quaternion : Subsystem
      mask help: normalize a quaternion
      mask Help:
      | Name:
      | 
      |     normalize_quaternion
      | 
      | Description:
      | 
      |     This block normalizes the quaternion q21. It should be used as a
      |     safety measure when computing quaternions.
      | 
      | Inputs  [size] [data type] [unit]:
      | 
      |     attitude quaternion q21  [4] [double] [-]
      | 
      | Outputs  [size] [data type] [unit]:
      | 
      |     normalized attitude quaternion q21  [4] [double] [-]
      mask Display: disp (' norm(q)')
  eom : Outport  VectorParamsAs1DForOutWhenUnconnected=off
  wires:
  normalize_quaternion/1(q_normalized) -> Bus Creator/3  "qIB"
  Reshape2/1 -> Bus Creator/6  "d_vBII"
  Reshape1/1 -> Bus Creator/5  "d_wBIB"
  Reshape/1 -> integration_eom/1  "d_x"
  d_pBII/1 -> Vector Concatenate/1
  d_vBII/1 -> Vector Concatenate/2, Reshape2/1
  d_qIB/1 -> Vector Concatenate/3
  d_wBIB/1 -> Vector Concatenate/4, Reshape1/1
  Vector Concatenate/1 -> Reshape/1  "d_x"
  integration_eom/1 -> Selector2/1, Selector3/1, Selector/1, Selector1/1  "x"
  x0/1 -> integration_eom/2
  Selector/1 -> Bus Creator/1  "pBII"
  Selector1/1 -> Bus Creator/2  "vBII"
  Selector2/1 -> normalize_quaternion/1(q)  "qIB"
  Selector3/1 -> Bus Creator/4  "wBIB"
  Bus Creator/1 -> eom/1  "eom_bus"

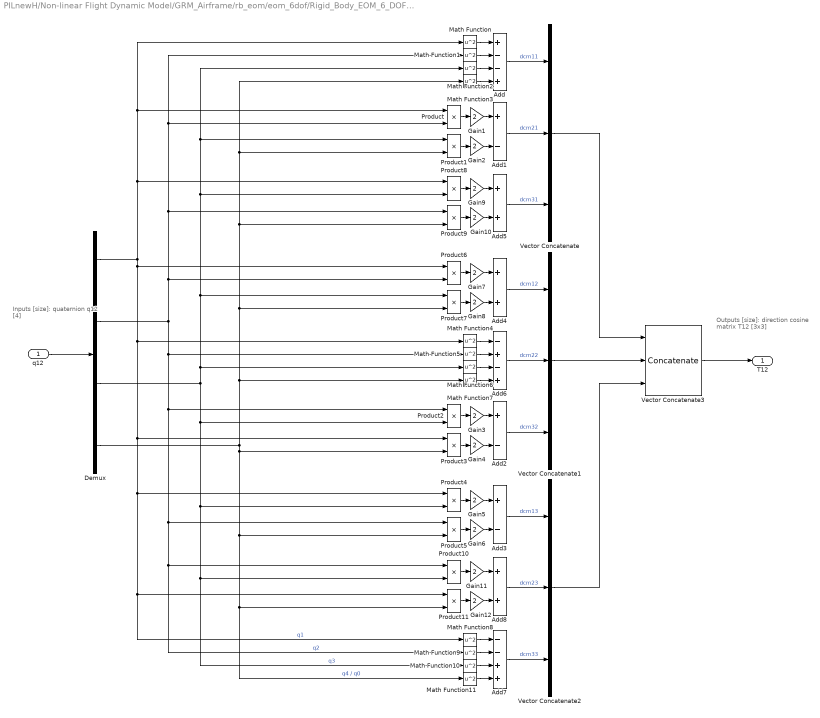
== system PILnewH/Non-linear Flight Dynamic Model/GRM_Airframe/rb_eom/eom_6dof/Rigid_Body_EOM_6_DOF/T12_from_q12 ==
  note: Inputs [size]:
      |
      | quaternion q12 [4]
  note: Outputs [size]:
      |
      | direction cosine matrix T12 [3x3]
  q12 : Inport  PortDimensions=4
  Add : Sum  Inputs=+--+
  Add1 : Sum  Inputs=+-
  Add2 : Sum  Inputs=+-
  Add3 : Sum  Inputs=+-
  Add4 : Sum
  Add5 : Sum
  Add6 : Sum  Inputs=-+-+
  Add7 : Sum  Inputs=--++
  Add8 : Sum
  Demux : Demux
  Gain{1..12} (12 alike) : Gain  Gain=2
  Math Function{,1..11} (12 alike) : Math  Operator=square  SignedPower=on  SaturateOnIntegerOverflow=on
  Product{,1..11} (12 alike) : Product
  Vector Concatenate : Concatenate  NumInputs=3
  Vector Concatenate1 : Concatenate  NumInputs=3
  Vector Concatenate2 : Concatenate  NumInputs=3
  Vector Concatenate3 : Concatenate  NumInputs=3  Mode=Multidimensional array  ConcatenateDimension=2
  T12 : Outport  PortDimensions=[3 3]  VectorParamsAs1DForOutWhenUnconnected=off
  wires:
  Product10/1 -> Gain11/1
  Product11/1 -> Gain12/1
  Gain11/1 -> Add8/1
  Gain12/1 -> Add8/2
  Math Function8/1 -> Add7/1
  Math Function9/1 -> Add7/2
  Math Function11/1 -> Add7/4
  Math Function10/1 -> Add7/3
  Math Function4/1 -> Add6/1
  Math Function5/1 -> Add6/2
  Math Function7/1 -> Add6/4
  Math Function6/1 -> Add6/3
  Product8/1 -> Gain9/1
  Product9/1 -> Gain10/1
  Gain9/1 -> Add5/1
  Gain10/1 -> Add5/2
  Product6/1 -> Gain7/1
  Product7/1 -> Gain8/1
  Gain7/1 -> Add4/1
  Gain8/1 -> Add4/2
  Product4/1 -> Gain5/1
  Product5/1 -> Gain6/1
  Gain5/1 -> Add3/1
  Gain6/1 -> Add3/2
  Product2/1 -> Gain3/1
  Product3/1 -> Gain4/1
  Gain3/1 -> Add2/1
  Gain4/1 -> Add2/2
  Gain2/1 -> Add1/2
  Gain1/1 -> Add1/1
  Product1/1 -> Gain2/1
  Product/1 -> Gain1/1
  Math Function3/1 -> Add/4
  Math Function2/1 -> Add/3
  Math Function1/1 -> Add/2
  Math Function/1 -> Add/1
  Add7/1 -> Vector Concatenate2/3  "dcm33"
  Add8/1 -> Vector Concatenate2/2  "dcm23"
  Add3/1 -> Vector Concatenate2/1  "dcm13"
  Add2/1 -> Vector Concatenate1/3  "dcm32"
  Add6/1 -> Vector Concatenate1/2  "dcm22"
  Add4/1 -> Vector Concatenate1/1  "dcm12"
  Add5/1 -> Vector Concatenate/3  "dcm31"
  Add1/1 -> Vector Concatenate/2  "dcm21"
  Add/1 -> Vector Concatenate/1  "dcm11"
  Vector Concatenate1/1 -> Vector Concatenate3/2
  Vector Concatenate2/1 -> Vector Concatenate3/3
  Vector Concatenate/1 -> Vector Concatenate3/1
  Vector Concatenate3/1 -> T12/1
  Demux/4 -> Product3/2, Product11/2, Math Function11/1, Product5/2, Math Function3/1, Product1/2, Product9/2, Product7/2, Math Function7/1  "q4 / q0"
  Demux/3 -> Math Function2/1, Product1/1, Product8/2, Product7/1, Math Function6/1, Product10/2, Math Function10/1, Product4/2, Product2/2  "q3"
  Demux/2 -> Math Function1/1, Product/2, Product9/1, Product6/2, Math Function5/1, Math Function9/1, Product10/1, Product5/1, Product2/1  "q2"
  Demux/1 -> Product6/1, Math Function4/1, Math Function8/1, Product11/1, Product4/1, Product3/1, Math Function/1, Product/1, Product8/1  "q1"
  q12/1 -> Demux/1

== system PILnewH/Non-linear Flight Dynamic Model/GRM_Airframe/rb_eom/eom_6dof/Rigid_Body_EOM_6_DOF/rb_eom_6dof ==
  note: d_wBIB = JBB \ (MBTB - d_JBB * wBIB - wBIB x (JBB*wBIB))
  FBTB : Inport
  mB : Inport  Port=2
  JBB : Inport  Port=3
  MBTB : Inport  Port=4
  d_JBB : Inport  Port=5
  qIB : Inport  Port=6
  vBII : Inport  Port=7
  wBIB : Inport  Port=8
  Divide : Product  Inputs=*/
  Divide1 : Product  Inputs=/*  Multiplication=Matrix(*)
  Product : Product  Multiplication=Matrix(*)
  Product1 : Product  Multiplication=Matrix(*)
  Saturation : Saturate  UpperLimit=Inf  LowerLimit=1e-6
      settings: AttributesFormatString=|
      | %<UpperLimit>
      | %<LowerLimit>
  Subtract : Sum  Inputs=+--
  calc_d_qIB : Subsystem
  cross_product : Subsystem
      mask help: cross product r3 = r1 x r2
      mask Help:
      | Name:
      | 
      |     cross_product
      | 
      | Description:
      | 
      |     This block implements the cross product r3 = r1 x r2.
      | 
      | Inputs  [size] [data type] [unit]:
      | 
      |     vector 1  [3] [double] [-]
      |     vector 2  [3] [double] [-]
      | 
      | Outputs  [size] [data type] [unit]:
      | 
      |     resulting vector  [3] [double] [-]
      mask Display: disp(' r3 = r1 x r2')
  r2_from_r1_trans_q21 : Subsystem
      mask help: transforms a vector from frame 1 to frame 2 by a quaternion
      mask Help:
      | Name:
      | 
      |     r2_from_r1_trans_q21
      | 
      | Description:
      | 
      |     This block implements the transformation of a vector from the frame 1
      |     to the frame 2 using the appropriate quaternion.
      | 
      | Inputs  [size] [data type] [unit]:
      | 
      |     vector in frame 1  [3] [double] [-]
      |     attitude quaternion q21  [4] [double] [-]
      | 
      | Outputs  [size] [data type] [unit]:
      | 
      |     vector in frame 2  [3] [double] [-]
      mask Display:
      | port_label('input', 1, 'r1')
      | port_label('input', 2, 'q21')
      | port_label('output', 1, 'r2')
      | disp('r_2 = q_{21} {\bf\cdot} r_1 {\bf\cdot} q_{21}^{\bf\prime}','texmode','on')
  d_pBII : Outport  VectorParamsAs1DForOutWhenUnconnected=off
  d_vBII : Outport  Port=2  VectorParamsAs1DForOutWhenUnconnected=off
  d_qIB : Outport  Port=3  VectorParamsAs1DForOutWhenUnconnected=off
  d_wBIB : Outport  Port=4  VectorParamsAs1DForOutWhenUnconnected=off
  wires:
  Saturation/1 -> Divide/2
  calc_d_qIB/1(d_qIB) -> d_qIB/1
  MBTB/1 -> Subtract/1
  Subtract/1 -> Divide1/2
  d_JBB/1 -> Product/1
  Product1/1 -> cross_product/2(r2)
  cross_product/1(r1_x_r2) -> Subtract/3
  Product/1 -> Subtract/2
  Divide1/1 -> d_wBIB/1
  wBIB/1 -> calc_d_qIB/2(wBIB), Product/2, cross_product/1(r1), Product1/2
  JBB/1 -> Divide1/1, Product1/1
  vBII/1 -> d_pBII/1
  r2_from_r1_trans_q21/1(r2) -> d_vBII/1  "aBII"
  qIB/1 -> calc_d_qIB/1(qIB), r2_from_r1_trans_q21/2(q21)
  Divide/1 -> r2_from_r1_trans_q21/1(r1)  "aBIB"
  mB/1 -> Saturation/1
  FBTB/1 -> Divide/1

== system PILnewH/Non-linear Flight Dynamic Model/GRM_Airframe/stream_flow/calc_stream_flow/Subsystem1/AoA_Sideslip_Alphatot_Phi ==
  note: Inputs [size]
      |
      | vector vBEB [3]
  note: Outputs [size]
      |
      | bus [4]
      | 	al  [1]
      | 	be [1]
      | 	th  [1]
      | 	fi   [1]
  note: falls a_vBEB == 0
      | Alle Winkel = 0
  vBEB : Inport
  Bus Creator : BusCreator  Inputs=4
  Constant : Constant  Value=[1; 0; 0; 1]
  Demux : Demux
  Demux1 : Demux  Outputs=3
  Divide : Product  Inputs=*/
  Divide1 : Product  Inputs=*/
  Switch : Switch  Criteria=u2 ~= 0
  Trigonometric Function : Trigonometry  Operator=atan2
  Trigonometric Function1 : Trigonometry  Operator=asin
  Trigonometric Function2 : Trigonometry  Operator=acos
  Trigonometric Function3 : Trigonometry  Operator=atan2
  Vector Concatenate : Concatenate  NumInputs=4
  norm_of_vector : Subsystem
      mask help: computes the norm of a vector
      mask Help:
      | Name:
      | 
      |     norm_of_vector
      | 
      | Description:
      | 
      |     This block computes the L2-norm (length) of a vector.
      | 
      | Inputs  [size] [data type] [unit]:
      | 
      |     vector  [3] [double] [-]
      | 
      | Outputs  [size] [data type] [unit]:
      | 
      |     norm of vector  [1] [double] [-]
      mask Display: disp (' norm(r) ')
  aero_angles : Outport  VectorParamsAs1DForOutWhenUnconnected=off
  wires:
  Demux1/2 -> Vector Concatenate/2  "vBEB_y"
  Demux1/3 -> Vector Concatenate/3  "vBEB_z"
  Demux1/1 -> Vector Concatenate/1  "vBEB_x"
  Divide1/1 -> Trigonometric Function2/1
  Trigonometric Function3/1 -> Bus Creator/4  "fi"
  Trigonometric Function2/1 -> Bus Creator/3  "th"
  Demux/4 -> Divide1/2, Divide/2  "a_vBEB"
  Switch/1 -> Demux/1
  Vector Concatenate/1 -> Switch/1
  Constant/1 -> Switch/3
  Bus Creator/1 -> aero_angles/1  "aero_angles_bus"
  norm_of_vector/1(norm_of_vector) -> Vector Concatenate/4, Switch/2  "a_vBEB"
  Trigonometric Function1/1 -> Bus Creator/2  "be"
  vBEB/1 -> norm_of_vector/1(vector), Demux1/1
  Demux/3 -> Trigonometric Function/1, Trigonometric Function3/2  "vBEB_z"
  Trigonometric Function/1 -> Bus Creator/1  "al"
  Divide/1 -> Trigonometric Function1/1
  Demux/1 -> Divide1/1, Trigonometric Function/2  "vBEB_x"
  Demux/2 -> Trigonometric Function3/1, Divide/1  "vBEB_y"

== system PILnewH/Non-linear Flight Dynamic Model/GRM_Airframe/stream_flow/calc_stream_flow/Subsystem1/calc_nondimensional_rates ==
  a_vB : Inport
  wBIB : Inport  Port=2
  Constant1 : Constant  Value=Aerodynamics.lref
      settings: AttributesFormatString=%<Value>
  Constant2 : Constant  Value=2
  Demux : Demux  Outputs=3
  Divide1 : Product  Inputs=/*/
  Product2 : Product
  Product3 : Product
  Product4 : Product
  Saturation1 : Saturate  UpperLimit=inf  LowerLimit=100*eps
      settings: AttributesFormatString=|
      | %<UpperLimit>
      | %<LowerLimit>
  Vector Concatenate : Concatenate  NumInputs=3
  wBIB_star : Outport  VectorParamsAs1DForOutWhenUnconnected=off
  wires:
  Demux/2 -> Product3/2
  Divide1/1 -> Product4/1, Product3/1, Product2/1
  Demux/3 -> Product4/2
  a_vB/1 -> Saturation1/1
  wBIB/1 -> Demux/1
  Product3/1 -> Vector Concatenate/2  "qBIB_star"
  Demux/1 -> Product2/2
  Saturation1/1 -> Divide1/1
  Constant1/1 -> Divide1/2
  Product4/1 -> Vector Concatenate/3  "rBIB_star"
  Product2/1 -> Vector Concatenate/1  "pBIB_star"
  Vector Concatenate/1 -> wBIB_star/1  "wBIB_star"
  Constant2/1 -> Divide1/3

== system PILnewH/Non-linear Flight Dynamic Model/GRM_Airframe/stream_flow/calc_stream_flow/Subsystem1/norm_of_vector ==
  note: Outputs [size]:
      |
      | norm of vector [1]
  note: Inputs [size]:
      |
      | vector  [3]
  vector : Inport
  Dot Product1 : DotProduct  InputSameDT=on  OutDataTypeStr=Inherit: Inherit via internal rule
  Math Function1 : Math  Operator=sqrt  SignedPower=on  SaturateOnIntegerOverflow=on
  norm_of_vector : Outport  VectorParamsAs1DForOutWhenUnconnected=off
  wires:
  vector/1 -> Dot Product1/1, Dot Product1/2
  Math Function1/1 -> norm_of_vector/1
  Dot Product1/1 -> Math Function1/1
